simulink model "flexiblelinksimulation"  (R2023a)
settings: Solver=ode45  StartTime=0.0  StopTime=1  MaxStep=1e-4  RelTol=1e-4
values from neighbouring files (symbols this model uses):
  gamma_2 = 0.1521*10^-10    (= 1.521e-11)    [flexiblelinkparams.m]    (also in spatialmode_symbolic_inverse.m = int(x*phi2, x, 0, L)/cf)
  I_b = 1.3549e-10    [flexiblelinkparams.m]
  I_h = 0.3    [flexiblelinkparams.m]    (also in flexiblelinksim.m)
  L = T - V    [acrobot_zerodynamics.m]    (also in flexiblelink_BVP.m = 1; flexiblelink_lagrange.m = 1/2 * (I_h + I_b) * dq1^2 + rho/2 * dq2^2 + rho * dq1 * dq2 ; flexiblelinkmodes.m = 1; flexiblelinkparams.m = 1)
  omega_2 = 32.5819    [flexiblelinkparams.m]
  phi2L = 1.7338e+08    (= 173380000)    [flexiblelinkparams.m]    (also in spatialmode_symbolic_inverse.m = subs(phi2,x,L))
  rho = 2700    [flexiblelinkmodes.m]    (also in flexiblelinkparams.m; flexiblelinksim.m; flexiblelinkvibration_FDM.m; spatialmode_numeric.m)
settings Model: Creator=MSI-  LastModifiedBy=MSI-

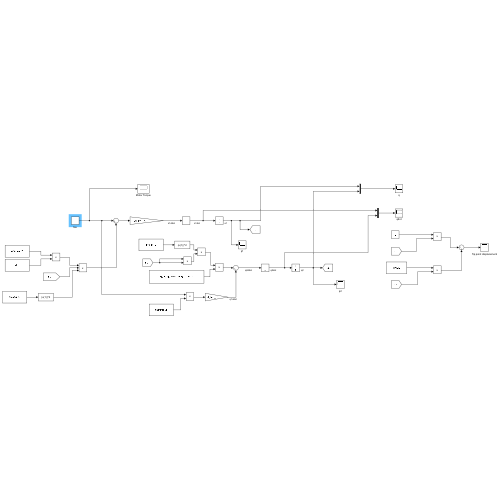
[thumbnail: Simulink's stored preview of the top-level diagram]
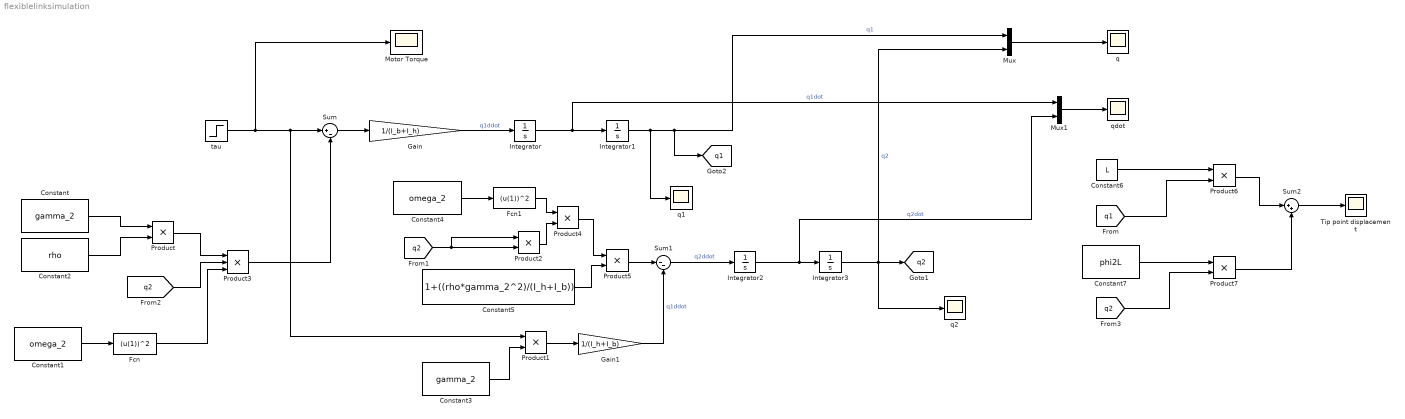
== system flexiblelinksimulation ==
  Constant : Constant  Value=gamma_2
  Constant1 : Constant  Value=omega_2
  Constant2 : Constant  Value=rho
  Constant3 : Constant  Value=gamma_2
  Constant4 : Constant  Value=omega_2
  Constant5 : Constant  Value=1+((rho*gamma_2^2)/(I_h+I_b))
  Constant6 : Constant  Value=L
  Constant7 : Constant  Value=phi2L
  Fcn : Fcn  Expr=(u(1))^2
  Fcn1 : Fcn  Expr=(u(1))^2
  Gain : Gain  Gain=1/(I_b+I_h)
  Gain1 : Gain  Gain=1/(I_h+I_b)
  Integrator{,1..3} (4 alike) : Integrator
  Motor Torque : Scope
  Mux : Mux  Inputs=2
  Mux1 : Mux  Inputs=2
  Product{,1..2,4..7} (7 alike) : Product
  Product3 : Product  Inputs=3
  Sum : Sum  Inputs=|+-
  Sum1 : Sum  Inputs=|--
  Sum2 : Sum  Inputs=|++
  Tip point displacement : Scope
  q : Scope
  q1 : Scope
  q2 : Scope
  qdot : Scope
  tau : Step  Before=0.25  After=0  SampleTime=0
  tag scope: q1=global, q2=global
  wires:
  Product3/1 -> Sum/2
  Constant2/1 -> Product/2
  Sum/1 -> Gain/1
  Constant/1 -> Product/1
  Gain/1 -> Integrator/1  "q1ddot"
  Integrator/1 -> Integrator1/1, Mux1/1  "q1dot"
  Integrator1/1 -> q1/1, [q1], Mux/1  "q1"
  tau/1 -> Motor Torque/1, Product1/1, Sum/1
  Constant3/1 -> Product1/2
  Product1/1 -> Gain1/1
  Integrator2/1 -> Mux1/2, Integrator3/1  "q2dot"
  Integrator3/1 -> q2/1, Mux/2, [q2]  "q2"
  [q2] -> Product2/1, Product2/2
  Sum1/1 -> Integrator2/1  "q2ddot"
  Product/1 -> Product3/1
  [q2] -> Product3/2
  Mux/1 -> q/1
  Mux1/1 -> qdot/1
  Constant1/1 -> Fcn/1
  Fcn/1 -> Product3/3
  Gain1/1 -> Sum1/2  "q1ddot"
  Constant4/1 -> Fcn1/1
  Fcn1/1 -> Product4/1
  Product2/1 -> Product4/2
  Product4/1 -> Product5/1
  Product5/1 -> Sum1/1
  Constant5/1 -> Product5/2
  Constant6/1 -> Product6/1
  [q2] -> Product7/2
  Constant7/1 -> Product7/1
  Product6/1 -> Sum2/1
  Product7/1 -> Sum2/2
  Sum2/1 -> Tip point displacement/1
  [q1] -> Product6/2
